simulink model "Part3BicycleSim"  (R2019a)
settings: Solver=VariableStepAuto  StartTime=0.0  StopTime=5  RelTol=1e-3
values from neighbouring files (symbols this model uses):
  A = [-c/ms c/ms;c/mu -c/mu]    [Part12b.m]    (also in Part33DofPar.m = [a11 a12 a13 a14; Part3BicyclePar.m = [-(caf+car)/(u*M) -((a*caf-b*car)/(u*M)+u); part23.m = [a11 a12 a13)
  a = 1.2    [Part33DofPar.m]    (also in Part3BicyclePar.m; part23.m)
  B = [-ks/ms ks/ms;ks/mu -ks/mu-kt/mu]    [Part12b.m]    (also in Part33DofPar.m = [b1;b2;b3;b4]; Part3BicyclePar.m = [caf/M;a*caf/Iz]; part23.m = [b1;b2;b4])
  b = 1.4    [Part33DofPar.m]    (also in Part3BicyclePar.m; part23.m)
  delta = 2.5/180*pi    (= 0.0436332312999)    [Part33DofPar.m]    (also in Part3BicyclePar.m)
libraries: simulink x1
settings Model: OrderedModelArguments=off  Creator=Ali  LastModifiedBy=a33shahi
settings DataIOCC: ReturnWorkspaceOutputs=off
settings DebuggingCC: PregeneratedLibrarySubsystemCodeDiagnostic=none  ArithmeticOperatorsInVariantConditions=warning
settings SFSimCC: SimUseLocalCustomCode=off
settings RTWCC: RTWUseLocalCustomCode=off

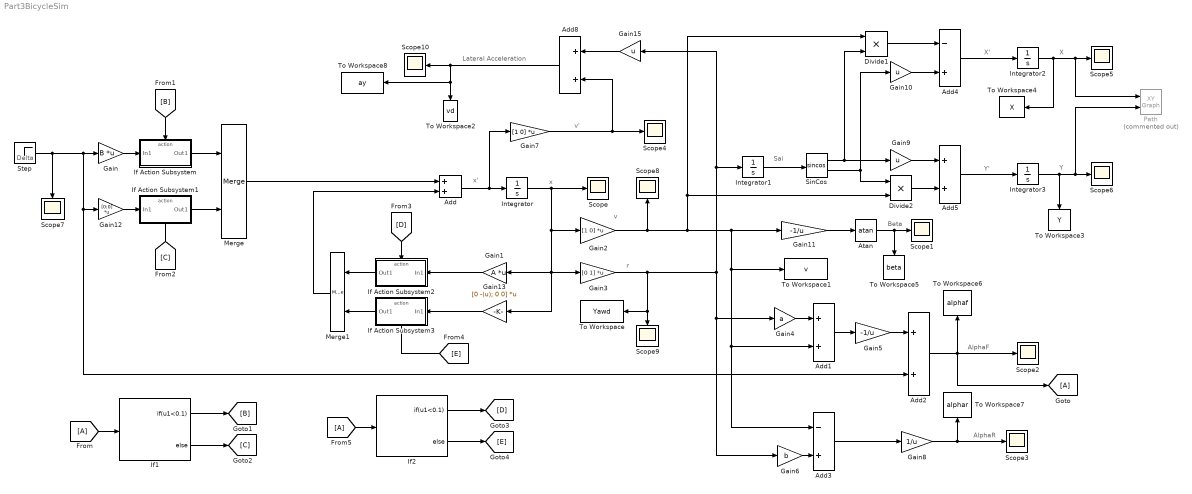
== system Part3BicycleSim ==
  note: Y
  note: Y'
  note: X
  note: X'
  note: Sai
  note: v'
  note: AlphaR
  note: AlphaF
  note: Beta
  note: r
  note: v
  note: x
  note: x'
  note: Delta
  note: Lateral Acceleration
  Add{,1..2,5,8} (5 alike) : Sum
  Add3 : Sum  Inputs=-+
  Add4 : Sum  Inputs=-+
  Atan : Trigonometry  Operator=atan
  Divide1 : Product  Inputs=**
  Divide2 : Product  Inputs=**
  Gain : Gain  Gain=B  Multiplication=Matrix(K*u)
  Gain1 : Gain  Gain=A  Multiplication=Matrix(K*u)
  Gain10 : Gain  Gain=u
  Gain11 : Gain  Gain=-1/u
  Gain12 : Gain  Gain=[0;0]  Multiplication=Matrix(K*u)
  Gain13 : Gain  Gain=[0 -(u); 0 0]  Multiplication=Matrix(K*u)
  Gain15 : Gain  Gain=u
  Gain2 : Gain  Gain=[1 0]  Multiplication=Matrix(K*u)
  Gain3 : Gain  Gain=[0 1]  Multiplication=Matrix(K*u)
  Gain4 : Gain  Gain=a
  Gain5 : Gain  Gain=-1/u
  Gain6 : Gain  Gain=b
  Gain7 : Gain  Gain=[1 0]  Multiplication=Matrix(K*u)
  Gain8 : Gain  Gain=1/u
  Gain9 : Gain  Gain=u
  If Action Subsystem : Subsystem  TreatAsAtomicUnit=on
  If Action Subsystem1 : Subsystem  TreatAsAtomicUnit=on
  If Action Subsystem2 : Subsystem  TreatAsAtomicUnit=on
  If Action Subsystem3 : Subsystem  TreatAsAtomicUnit=on
  If1 : If  IfExpression=u1<0.1
  If2 : If  IfExpression=u1<0.1
  Integrator{,1..3} (4 alike) : Integrator
  Merge : Merge
  Merge1 : Merge
  Path : simulink/Sinks/XY Graph  Commented=on  xmin=-100  xmax=200  ymin=-100  ymax=200  st=-1
  Scope{,1..10} (11 alike) : Scope
  SinCos : Trigonometry  Operator=sincos
  Step : Step  Time=0  After=delta  SampleTime=0
  To Workspace : ToWorkspace  VariableName=Yawd  SaveFormat=Timeseries  SampleTime=-1
  To Workspace1 : ToWorkspace  VariableName=v  SaveFormat=Timeseries  SampleTime=-1
  To Workspace2 : ToWorkspace  VariableName=vd  SaveFormat=Timeseries  SampleTime=-1
  To Workspace3 : ToWorkspace  VariableName=Y  SaveFormat=Timeseries  SampleTime=-1
  To Workspace4 : ToWorkspace  VariableName=X  SaveFormat=Timeseries  SampleTime=-1
  To Workspace5 : ToWorkspace  VariableName=beta  SaveFormat=Timeseries  SampleTime=-1
  To Workspace6 : ToWorkspace  VariableName=alphaf  SaveFormat=Timeseries  SampleTime=-1
  To Workspace7 : ToWorkspace  VariableName=alphar  SaveFormat=Timeseries  SampleTime=-1
  To Workspace8 : ToWorkspace  VariableName=ay  SaveFormat=Timeseries  SampleTime=-1
  wires:
  Add/1 -> Gain7/1, Integrator/1
  Gain3/1 -> Scope9/1, To Workspace/1, Gain15/1, Integrator1/1, Gain4/1, Gain6/1
  Atan/1 -> To Workspace5/1, Scope1/1
  Gain4/1 -> Add1/1
  Add1/1 -> Gain5/1
  Gain5/1 -> Add2/1
  Gain6/1 -> Add3/2
  Add3/1 -> Gain8/1
  Gain7/1 -> Add8/2, Scope4/1
  Integrator1/1 -> SinCos/1
  Gain8/1 -> Scope3/1, To Workspace7/1
  SinCos/2 -> Divide2/1, Gain10/1
  Gain10/1 -> Add4/2
  SinCos/1 -> Gain9/1, Divide1/2
  Gain2/1 -> Scope8/1, Divide2/2, Divide1/1, To Workspace1/1, Add3/1, Add1/2, Gain11/1
  Divide1/1 -> Add4/1
  Add4/1 -> Integrator2/1
  Integrator2/1 -> To Workspace4/1, Path/1, Scope5/1
  Gain9/1 -> Add5/1
  Divide2/1 -> Add5/2
  Integrator3/1 -> To Workspace3/1, Path/2, Scope6/1
  Add5/1 -> Integrator3/1
  Gain11/1 -> Atan/1
  Add8/1 -> To Workspace2/1, To Workspace8/1, Scope10/1
  Gain15/1 -> Add8/1
  Step/1 -> Scope7/1, Gain/1, Add2/2, Gain12/1
  Add2/1 -> [A], Scope2/1, To Workspace6/1
  [A] -> If1/1
  If1/1 -> [B]
  [B] -> If Action Subsystem/Action
  If1/2 -> [C]
  Merge/1 -> Add/1
  [C] -> If Action Subsystem1/Action
  If Action Subsystem/1(Out1) -> Merge/1
  Gain/1 -> If Action Subsystem/1(In1)
  Gain12/1 -> If Action Subsystem1/1(In1)
  If Action Subsystem1/1(Out1) -> Merge/2
  [D] -> If Action Subsystem2/Action
  Gain1/1 -> If Action Subsystem2/1(In1)
  If Action Subsystem2/1(Out1) -> Merge1/1
  Merge1/1 -> Add/2
  [E] -> If Action Subsystem3/Action
  Integrator/1 -> Gain13/1, Gain1/1, Gain3/1, Gain2/1, Scope/1
  Gain13/1 -> If Action Subsystem3/1(In1)
  If Action Subsystem3/1(Out1) -> Merge1/2
  If2/2 -> [E]
  If2/1 -> [D]
  [A] -> If2/1

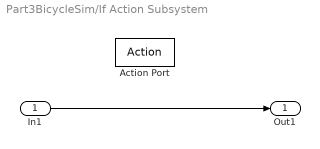
== system Part3BicycleSim/If Action Subsystem ==
  In1 : Inport
  Action Port : ActionPort  ActionPortLabel=if(u1<0.1)
  Out1 : Outport
  wires:
  In1/1 -> Out1/1

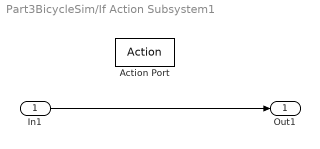
== system Part3BicycleSim/If Action Subsystem1 ==
  In1 : Inport
  Action Port : ActionPort  ActionPortLabel=else
  Out1 : Outport
  wires:
  In1/1 -> Out1/1

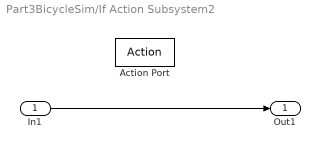
== system Part3BicycleSim/If Action Subsystem2 ==
  In1 : Inport
  Action Port : ActionPort  ActionPortLabel=if(u1<0.1)
  Out1 : Outport
  wires:
  In1/1 -> Out1/1

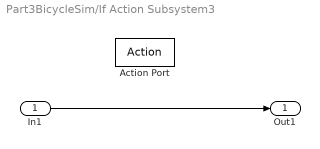
== system Part3BicycleSim/If Action Subsystem3 ==
  In1 : Inport
  Action Port : ActionPort  ActionPortLabel=else
  Out1 : Outport
  wires:
  In1/1 -> Out1/1
